simulink model "singleDPD"  (R2023a)
settings: Solver=FixedStepAuto  StartTime=0.0  StopTime=5*Tstep*ofdmSymLen*6  RelTol=1e-3
PreLoadFcn:
  | %{
  | % 100 MHz scenario
  | % scs = 30e3;
  | % fftLength = 4096;
  | % NSubcarriers = 3276;
  | % cpLength = 288;
  | % windowLength = 20;
  | 
  | % 5 MHz scenario
  | scs = 30e3;
  | fftLength = 256;
  | NSubcarriers = 132;
  | cpLength = 18;
  | windowLength = 6;
  | 
  | nGuardBandCarrier = fftLength - NSubcarriers;
  | ofdmSymLen = fftLength+cpLength;
  | overSamplingRate = 7;
  | filterLength = 6*70;
  | 
  | BW = scs*fftLength;                       %  Signal BW
  | Tstep = 1/BW;                   %  Simulation BW BB
  | RF = 3.7e9;                       %  RF center frequency
  | IF = 500e6;                          % IF frequency
  | dataRatePA = 1/BW;  % PA characterization sample time
  | N = nGuardBandCarrier/2;
  | HPF_cutoff = RF - 500e6;
  | 
  | bw = 5e6; %100e6;
  | [txWaveform, sampleRate] = helperPACharGenerateOFDM(bw);
  | 
  | dataFileName = sprintf("helperPACharSavedData%dMHz",bw/1e6);
  | load(dataFileName,"results")
  | paInput = results.InputWaveform;
  | paOutput = results.OutputWaveform;
  | modType = 'memPoly';
  | memLen = 5;
  | degLen = 5;
  | halfDataPts = round(length(paInput)/2);
  | origState = warning;
  | warning('off', 'MATLAB:rankDeficientMatrix')
  | paModelMemPoly = double(helperPACharMemPolyModel('coefficientFinder', ...
  |   paInput(1:halfDataPts),paOutput(1:halfDataPts),memLen,degLen,modType));
  | warning(origState);
  | 
  | gain = results.LinearGain;
  | scaleFactor = double(max(abs(paOutput))/max(abs(txWaveform))/gain);
  | %}
InitFcn:
  | % 100 MHz scenario
  |  scs = 30e3;
  |  fftLength = 4096;
  |  NSubcarriers = 3276;
  |  cpLength = 288;
  |  windowLength = 20;
  | 
  | % 5 MHz scenario
  | %scs = 30e3; % Subcarrier spacing
  | %fftLength = 256;
  | %NSubcarriers = 132;
  | %cpLength = 18; % cyclic prefix length
  | %windowLength = 6;
  | 
  | nGuardBandCarrier = fftLength - NSubcarriers;
  | ofdmSymLen = fftLength+cpLength;
  | overSamplingRate = 7;
  | filterLength = 6*70;
  | 
  | BW = scs*fftLength;                       %  Signal BW
  | Tstep = 1/BW;                   %  Simulation BW BB
  | RF = 1e9; %3.7e9;                       %  RF center frequency
  | IF = 500e6;                          % IF frequency
  | dataRatePA = 1/BW;  % PA characterization sample time
  | N = nGuardBandCarrier/2;
  | HPF_cutoff = RF - 500e6;
  | 
  | bw = 5e6; %100e6;
  | [txWaveform, sampleRate] = helperPACharGenerateOFDM(bw);
  | 
  | dataFileName = sprintf("helperPACharSavedData%dMHz",bw/1e6);
  | dataFileName = "helperPACharSavedData100MHz"
  | load(dataFileName,"results")
  | paInput = results.InputWaveform;
  | paOutput = results.OutputWaveform;
  | modType = 'memPoly';
  | memLen = 5;
  | degLen = 5;
  | halfDataPts = round(length(paInput)/2);
  | origState = warning;
  | warning('off', 'MATLAB:rankDeficientMatrix')
  | paModelMemPoly = double(helperPACharMemPolyModel('coefficientFinder', ...
  |   paInput(1:halfDataPts),paOutput(1:halfDataPts),memLen,degLen,modType));
  | warning(origState);
  | 
  | gain = results.LinearGain;
  | scaleFactor = double(max(abs(paOutput))/max(abs(txWaveform))/gain);
undefined symbols (not defined in the file or in its folder): hpaGain, S
libraries: simrfV2elements x20, simrfV2util1 x11, dspstat3 x8, simrfV2systems x3, simrfV2_lib x3, commofdm x2, simrfV2junction1 x2, commrfcorlib x2, simulink x2, commrandsrc3 x1, commdigbbndam3 x1, commutil2 x1
Description:
  | Power Amplifier Characterization with DPD for Reduced Signal Distortion
settings Model: SimulationMode=accelerator  Creator=The MathWorks, Inc.  LastModifiedBy=Hossein
settings SolverCC: ZeroCrossAlgorithm=Adaptive  AlgebraicLoopSolver=TrustRegion
settings DataIOCC: LimitDataPoints=on  SaveFormat=Array  SaveOutput=off  SignalLogging=off  DSMLogging=off  SaveTime=off  ReturnWorkspaceOutputs=off
settings OptimizationCC: BlockReduction=off  BooleanDataType=off  ReuseModelBlockBuffer=off  LifeSpan=inf
settings DebuggingCC: SaveWithParameterizedLinksMsg=none  UnderspecifiedInitializationDetection=Classic  MergeDetectMultiDrivingBlocksExec=none  SignalResolutionControl=TryResolveAllWithWarning  UnconnectedInputMsg=warning  UnconnectedOutputMsg=warning  UnconnectedLineMsg=warning  AllowSymbolicDim=off  SFUnexpectedBacktrackingDiag=warning  SFNoUnconditionalDefaultTransitionDiag=warning  SFExecutionAtInitializationDiag=none  ArithmeticOperatorsInVariantConditions=warning
settings HardwareCC: ProdBitPerPointer=32  ProdBitPerSizeT=32  ProdBitPerPtrDiffT=32  ProdLargestAtomicFloat=None  ProdIntDivRoundTo=Undefined  ProdEndianess=Unspecified  ProdWordSize=32  ProdHWDeviceType=32-bit Generic  TargetBitPerPointer=64  TargetBitPerSizeT=64  TargetBitPerPtrDiffT=64  TargetLongLongMode=on  TargetIntDivRoundTo=Zero  TargetEndianess=LittleEndian  TargetWordSize=64  TargetHWDeviceType=MATLAB Host  ProdEqTarget=off
settings ModelReferenceCC: EnableRefExpFcnMdlSchedulingChecks=on  PropagateSignalLabelsOutOfModel=off
settings SFSimCC: SimUseLocalCustomCode=off
settings RTWCC: RTWUseLocalCustomCode=off  BuildConfiguration=Faster Runs  DLArmComputeVersion=19.05
settings CodeAppCC: StateflowObjectComments=on
settings GRTTargetCC: TargetLangStandard=C89/C90 (ANSI)
settings ConfigComp: CovMetricSettings=dw  CovSaveCumulativeToWorkspaceVar=on  CovSaveSingleToWorkspaceVar=on  CovExternalEMLEnable=off
settings SimscapeCC: SimscapeNormalizeSystem=off

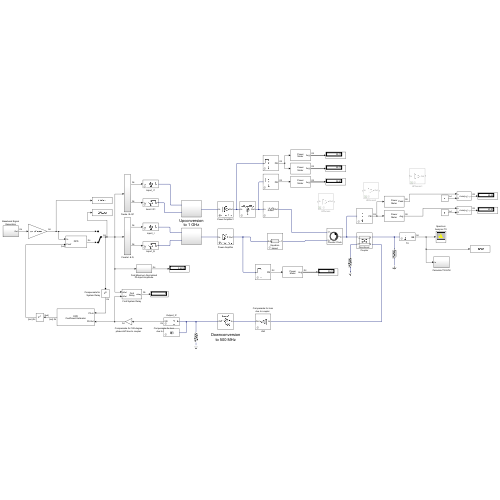
[thumbnail: Simulink's stored preview of the top-level diagram]
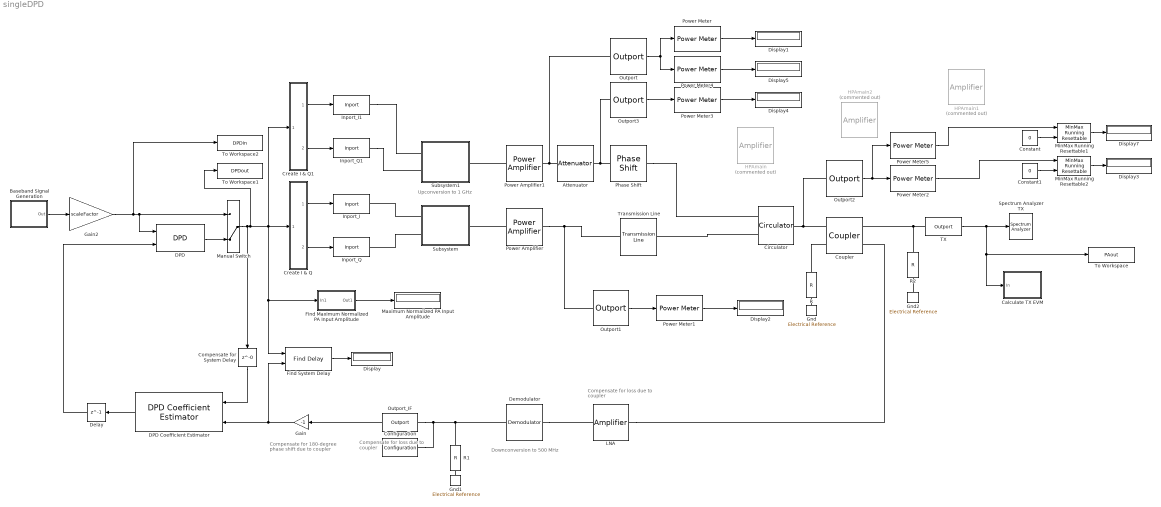
== system singleDPD ==
  note: Upconversion
      | to 1 GHz
  note: Compensate for loss
      | due to coupler
  note: Compensate for 180-degree
      | phase shift due to coupler
  note: Downconversion
      | to 500 MHz
  note: Compensate for loss
      | due to coupler
  Attenuator : simrfV2elements/Attenuator  classname=attenuator  Att=2.5  Zin=50  Zout=50  AddNoise=on  InternalGrounding=on
  Baseband Signal Generation : Subsystem
  Calculate TX EVM : Subsystem
  Circulator : simrfV2junction1/Circulator  classname=circulators  DataSource=Network-parameters  NumPorts=3  DeviceCirculator=Circulator counter clockwise  DeviceDivider=T power divider  DeviceCoupler=Directional coupler  Paramtype=S-parameters  Sparam=[0 0 1; 1 0 0; 0 1 0]  SparamFreq=1e9 Hz  SparamZ0=50  Phase12=0  Phase33=0  Alpha=0  NumberDividerOutports=2  Coupling=0  Directivity=inf  InsertionLoss=inf  ReturnLoss=inf  InternalGrounding=on  SparamRepresentation=Frequency domain  FitOpt=Share all poles  FitTol=-40  MaxPoles=48
  Compensate for System Delay : Delay  DelayLength=0
  Configuration : simrfV2util1/Configuration  AutoFreq=on  Tones="[3.2         3.7] GHz"  Harmonics="[5  5]"  NormalizeCarrierPower=on  SolverType=Auto  UseCCode=on  StepSize=Tstep/overSamplingRate s  AddNoise=on  defaultRNG=on  Seed=0  Temperature=290.0 K  SolverDelFlag=0  AbsTol=1e-6  RelTol=1e-3  MaxIter=10  ErrorEstimationType=2-norm over all variables  EnableInterpFilter=off  HiddenFIRfilterControllerParam=off  SmallSignalApprox=off  AllSimFreqs=on  SimFreqs=[] Hz  SimFreqsInternal=[]  SamplesPerFrame=1
  Constant : Constant  Value=0
  Constant1 : Constant  Value=0
  Coupler : simrfV2junction1/Coupler  classname=couplers  DataSource=Network-parameters  NumPorts=4  DeviceCirculator=Circulator clockwise  DeviceDivider=T power divider  DeviceCoupler=Directional coupler  Paramtype=S-parameters  Sparam=[0 0 1; 1 0 0; 0 1 0]  SparamFreq=1e9 Hz  SparamZ0=50  Phase12=0  Phase33=0  Alpha=0  NumberDividerOutports=2  Coupling=55  Directivity=inf  InsertionLoss=0.0001  ReturnLoss=inf  InternalGrounding=on  SparamRepresentation=Frequency domain  FitOpt=Share all poles  FitTol=-40  MaxPoles=48
  Create I & Q : Subsystem
  Create I & Q1 : Subsystem
  DPD : commrfcorlib/DPD  PolynomialType=Memory polynomial  CoefficientSource=Input port  Coefficients=complex([1 0 0 0 0; 0 0 0 0 0; 0 0 0 0 0])  SimulateUsing=Code generation
  DPD Coefficient Estimator : commrfcorlib/DPD Coefficient Estimator  DesiredAmplitudeGaindB=10*log10(gain)  PolynomialType=Memory polynomial  Degree=6  MemoryDepth=5  Algorithm=Recursive least squares  ForgettingFactorSource=Property  ForgettingFactor=0.999  InitialCoefficientEstimate=[]  SimulateUsing=Code generation
  Delay : Delay  DelayLength=1
  Demodulator : simrfV2systems/Demodulator  classname=rfdemod  Source_linear_gain=Available power gain  linear_gain=0 dB  Poly_Coeffs=[0 1]  LOFreq=RF-IF Hz  Zin=50  Zout=50  AddIRFilter=on  AddCSFilter=off  InternalGrounding=on  ForceNextInit=off  Source_Poly=Even and odd order  IPType=Input  IP2=inf dBm  IP3=inf dBm  P1dB=inf dBm  Psat=inf dBm  Gcomp=inf dBm  NF=1  Isolation=inf dB  AddPhaseNoise=off  PhaseNoiseOffset=[5e5 1e6 5e6]  PhaseNoiseLevel=[-108 -130 -140]  AutoImpulseLengthPN=on  ImpulseLengthPN=1e-10  ImpulseLength_unitPN=s  DesignMethodIR=Ideal  ResponseTypeIR=Highpass  ImplementationIR=LC Tee  ImplementationIdealIR=Constant per carrier  ImplementationRationalIR=Transfer function  UseFilterOrderIR=on  FilterOrderIR=3  PassFreq_lpIR=1  PassFreq_lp_unitIR=GHz  PassFreq_hpIR=HPF_cutoff  PassFreq_hp_unitIR=Hz  PassFreq_bpIR=[2 3]  PassFreq_bp_unitIR=GHz  PassFreq_bsIR=[1 4]  PassFreq_bs_unitIR=GHz  PassAttenIR=10*log10(2)  StopFreq_lpIR=2  StopFreq_lp_unitIR=GHz  StopFreq_hpIR=1  StopFreq_hp_unitIR=GHz  StopFreq_bpIR=[1.5 3.5]  StopFreq_bp_unitIR=GHz  StopFreq_bsIR=[2.1 2.9]  StopFreq_bs_unitIR=GHz  StopAttenIR=40  RsrcIR=50  RloadIR=50  AutoImpulseLengthIR=on  ImpulseLengthIR=1e-10  ImpulseLength_unitIR=s  DesignMethodCS=Ideal  ResponseTypeCS=Lowpass  ImplementationCS=LC Tee  ImplementationIdealCS=Constant per carrier  ImplementationRationalCS=Transfer function  UseFilterOrderCS=on  FilterOrderCS=3  PassFreq_lpCS=1  PassFreq_lp_unitCS=GHz  PassFreq_hpCS=2  PassFreq_hp_unitCS=GHz  PassFreq_bpCS=[2 3]  PassFreq_bp_unitCS=GHz  PassFreq_bsCS=[1 4]  PassFreq_bs_unitCS=GHz  PassAttenCS=10*log10(2)  StopFreq_lpCS=2  StopFreq_lp_unitCS=GHz  StopFreq_hpCS=1  StopFreq_hp_unitCS=GHz  StopFreq_bpCS=[1.5 3.5]  StopFreq_bp_unitCS=GHz  StopFreq_bsCS=[2.1 2.9]  StopFreq_bs_unitCS=GHz  StopAttenCS=40  RsrcCS=50  RloadCS=50  AutoImpulseLengthCS=on  ImpulseLengthCS=1e-10  ImpulseLength_unitCS=s
  Display{,1..5,7} (7 alike) : Display
  Find Maximum Normalized PA Input Amplitude : Subsystem
  Find System Delay : commutil2/Find Delay  corrLength=200  chgSigOP=off  stopUpdate=off  numConstDelay=3
  Gain : Gain  Gain=-1
  Gain2 : Gain  Gain=scaleFactor
  Gnd : simrfV2_lib/Elements/Electrical Reference
      settings: InternalSimscapePortConfiguration="{\"Bottom\":[],\"Left\":[{\"id\":\"V\",\"label\":\"\",\"type\":\"foundation.rf.circuitenvelope\"}],\"Right\":[],\"Top\":[]}"
  Gnd1 : simrfV2_lib/Elements/Electrical Reference
      settings: InternalSimscapePortConfiguration="{\"Bottom\":[],\"Left\":[{\"id\":\"V\",\"label\":\"\",\"type\":\"foundation.rf.circuitenvelope\"}],\"Right\":[],\"Top\":[]}"
  Gnd2 : simrfV2_lib/Elements/Electrical Reference
      settings: InternalSimscapePortConfiguration="{\"Bottom\":[],\"Left\":[{\"id\":\"V\",\"label\":\"\",\"type\":\"foundation.rf.circuitenvelope\"}],\"Right\":[],\"Top\":[]}"
  HPAmain : simrfV2elements/Amplifier  Commented=on  classname=amplifier  DataSource=Network-parameters  File=unitygain.s2p  isNetworkObj=off  Paramtype=S-parameters  Sparam=0  SparamFreq=CarrierFreq GHz  SparamZ0=50  isRationalObj=off  Residues=0  Poles=0  DF={0 0; 1 0}  Source_linear_gain=Available power gain  linear_gain=hpaGain - 3.5 dB  AmAmAmPmTable=[-25,5,-1;-10,20,-2;0,27,5;5,28,12]  Zin=50  Zout=50  Source_Poly=Odd order  Poly_Coeffs=[0 1]  IPType=Output  IP2=inf dBm  IP3=hpaIP3 dBm  P1dB=hpaP1dB dBm  Psat=inf dBm  Gcomp=inf dBm  InternalGrounding=on  SourceFreq=Extracted from data source  PlotFreq=1 Hz  PlotType=X-Y plane  YParam1=S(2,1)  YFormat1=Magnitude (dB)  YParam2=None  YFormat2=Magnitude (dB)  YOption=Linear  XOption=Linear  SparamRepresentation=Frequency domain  FitTol=-40  FitOpt=Fit individually  MaxPoles=48  AutoImpulseLength=off  ImpulseLength=0 s  MagModeling=off  AddNoise=on  NoiseType=Noise figure  NoiseDist=White  NF=hpaNF  MinNF=0  Gopt=0  RN=0  CarrierFreq=0 Hz  NoiseAutoImpulseLength=on  NoiseImpulseLength=1e-10 s  ConstS21NL=on  OpFreq=0 Hz  SetOpFreqAsMaxS21=on
  HPAmain1 : simrfV2elements/Amplifier  Commented=on  classname=amplifier  DataSource=Network-parameters  File=unitygain.s2p  isNetworkObj=off  Paramtype=S-parameters  Sparam=0  SparamFreq=CarrierFreq GHz  SparamZ0=50  isRationalObj=off  Residues=0  Poles=0  DF={0 0; 1 0}  Source_linear_gain=Available power gain  linear_gain=10 dB  AmAmAmPmTable=[-25,5,-1;-10,20,-2;0,27,5;5,28,12]  Zin=50  Zout=50  Source_Poly=Odd order  Poly_Coeffs=[0 1]  IPType=Output  IP2=inf dBm  IP3=48 dBm  P1dB=40 dBm  Psat=45 dBm  Gcomp=inf dBm  InternalGrounding=on  SourceFreq=Extracted from data source  PlotFreq=1 Hz  PlotType=X-Y plane  YParam1=S(2,1)  YFormat1=Magnitude (dB)  YParam2=None  YFormat2=Magnitude (dB)  YOption=Linear  XOption=Linear  SparamRepresentation=Frequency domain  FitTol=-40  FitOpt=Fit individually  MaxPoles=48  AutoImpulseLength=off  ImpulseLength=0 s  MagModeling=off  AddNoise=on  NoiseType=Noise figure  NoiseDist=White  NF=0  MinNF=0  Gopt=0  RN=0  CarrierFreq=0 Hz  NoiseAutoImpulseLength=on  NoiseImpulseLength=1e-10 s  ConstS21NL=on  OpFreq=0 Hz  SetOpFreqAsMaxS21=on
  HPAmain2 : simrfV2elements/Amplifier  Commented=on  classname=amplifier  DataSource=Network-parameters  File=unitygain.s2p  isNetworkObj=off  Paramtype=S-parameters  Sparam=0  SparamFreq=CarrierFreq GHz  SparamZ0=50  isRationalObj=off  Residues=0  Poles=0  DF={0 0; 1 0}  Source_linear_gain=Available power gain  linear_gain=10 dB  AmAmAmPmTable=[-25,5,-1;-10,20,-2;0,27,5;5,28,12]  Zin=50  Zout=50  Source_Poly=Odd order  Poly_Coeffs=[0 1]  IPType=Output  IP2=inf dBm  IP3=48 - 3.5 dBm  P1dB=40 - 3.5 dBm  Psat=45 - 3.5 dBm  Gcomp=inf dBm  InternalGrounding=on  SourceFreq=Extracted from data source  PlotFreq=1 Hz  PlotType=X-Y plane  YParam1=S(2,1)  YFormat1=Magnitude (dB)  YParam2=None  YFormat2=Magnitude (dB)  YOption=Linear  XOption=Linear  SparamRepresentation=Frequency domain  FitTol=-40  FitOpt=Fit individually  MaxPoles=48  AutoImpulseLength=off  ImpulseLength=0 s  MagModeling=off  AddNoise=on  NoiseType=Noise figure  NoiseDist=White  NF=0  MinNF=0  Gopt=0  RN=0  CarrierFreq=0 Hz  NoiseAutoImpulseLength=on  NoiseImpulseLength=1e-10 s  ConstS21NL=on  OpFreq=0 Hz  SetOpFreqAsMaxS21=on
  Inport_I : simrfV2util1/Inport  SimulinkInputSignalType=Ideal voltage  CarrierFreq=0 Hz  ZS=0  UseSqWave=off  NumCoeff=10  Bias=0  DutyCyc=50  InternalGrounding=on
  Inport_I1 : simrfV2util1/Inport  SimulinkInputSignalType=Ideal voltage  CarrierFreq=0 Hz  ZS=0  UseSqWave=off  NumCoeff=10  Bias=0  DutyCyc=50  InternalGrounding=on
  Inport_Q : simrfV2util1/Inport  SimulinkInputSignalType=Ideal voltage  CarrierFreq=0 Hz  ZS=0  UseSqWave=off  NumCoeff=10  Bias=0  DutyCyc=50  InternalGrounding=on
  Inport_Q1 : simrfV2util1/Inport  SimulinkInputSignalType=Ideal voltage  CarrierFreq=0 Hz  ZS=0  UseSqWave=off  NumCoeff=10  Bias=0  DutyCyc=50  InternalGrounding=on
  LNA : simrfV2elements/Amplifier  classname=amplifier  DataSource=Data file  File=unitygain.s2p  isNetworkObj=off  Paramtype=S-parameters  Sparam=[0 0;1 0]  SparamFreq=1e9 Hz  SparamZ0=50  isRationalObj=off  Residues=0  Poles=0  DF={0 0; 1 0}  Source_linear_gain=Available power gain  linear_gain=55 dB  AmAmAmPmTable=[-25,5,-1;-10,20,-2;0,27,5;5,28,12]  Zin=50  Zout=50  Source_Poly=Odd order  Poly_Coeffs=[0 1]  IPType=Output  IP2=19.5 dBm  IP3=inf dBm  P1dB=inf dBm  Psat=inf dBm  Gcomp=inf dBm  InternalGrounding=on  SourceFreq=Extracted from data source  PlotFreq=0 Hz  PlotType=X-Y plane  YParam1=S(1,1)  YFormat1=Magnitude (dB)  YParam2=None  YFormat2=Magnitude (dB)  YOption=Linear  XOption=Linear  SparamRepresentation=Time domain (rationalfit)  FitTol=-40  FitOpt=Share all poles  MaxPoles=48  AutoImpulseLength=off  ImpulseLength=0 s  MagModeling=off  AddNoise=on  NoiseType=Noise figure  NoiseDist=White  NF=0.1  MinNF=0  Gopt=0  RN=0  CarrierFreq=0 Hz  NoiseAutoImpulseLength=on  NoiseImpulseLength=1e-10 s  ConstS21NL=on  OpFreq=0 Hz  SetOpFreqAsMaxS21=on
  Manual Switch : ManualSwitch  CurrentSetting=0
  Maximum Normalized PA Input Amplitude : Display
  MinMax Running Resettable1 : simulink/Math Operations/MinMax Running Resettable  Function=max  vinit=0.0
  MinMax Running Resettable2 : simulink/Math Operations/MinMax Running Resettable  Function=max  vinit=0.0
  Outport{,1..3} (4 alike) : simrfV2util1/Outport  SensorType=Ideal voltage  OutputFormat=Real Passband  CarrierFreq=RF Hz  ZL=Inf  InternalGrounding=on  StepSize=1e-6 s  AutoStep=on  HalfPolyphaseLength=12
  Outport_IF : simrfV2util1/Outport  SensorType=Ideal voltage  OutputFormat=Complex Baseband  CarrierFreq=IF Hz  ZL=Inf  InternalGrounding=on  StepSize=-1 s  AutoStep=off  HalfPolyphaseLength=0
  Phase Shift : simrfV2elements/Phase Shift  PhaseShift=90 deg  InternalGrounding=on
  Power Amplifier : simrfV2elements/Power Amplifier  classname=poweramp  ModelType=Memory polynomial  CoeffMatrix=paModelMemPoly  UnitDelay=dataRatePA/overSamplingRate  Rin=50  Rout=50  InternalGrounding=on
  Power Amplifier1 : simrfV2elements/Power Amplifier  classname=poweramp  ModelType=Memory polynomial  CoeffMatrix=paModelMemPoly  UnitDelay=dataRatePA/overSamplingRate  Rin=50  Rout=50  InternalGrounding=on
  Power Meter{,1,3..4} (4 alike) : dspstat3/Power Meter  Measurement=Average power  ReferenceLoad=50  OutputPowerUnits=dBm  WindowLength=2048  OverlapLength=2047  AllowArbitraryInputLength=on  ComputeCCDF=off  PowerRange=50  PowerResolution=0.1  CCDFOutput=Relative power (dB above average power)  ProbabilityVector=[ 10; 1; 0.1; 0.01; 0.001; 0.0001 ]  RelativePowerVector=[ 0; 3; 6; 9; 12 ]  ResetPort=off  SimulateUsing=Code generation
      settings: LibrarySourceBlock=commutil2/Power Meter
  Power Meter2 : dspstat3/Power Meter  Measurement=Average power  ReferenceLoad=50  OutputPowerUnits=dBm  WindowLength=2048*2  OverlapLength=2047*2+1  AllowArbitraryInputLength=off  ComputeCCDF=off  PowerRange=50  PowerResolution=0.1  CCDFOutput=Relative power (dB above average power)  ProbabilityVector=[ 10; 1; 0.1; 0.01; 0.001; 0.0001 ]  RelativePowerVector=[ 0; 3; 6; 9; 12 ]  ResetPort=off  SimulateUsing=Code generation
      settings: LibrarySourceBlock=commutil2/Power Meter
  Power Meter5 : dspstat3/Power Meter  Measurement=Peak power  ReferenceLoad=50  OutputPowerUnits=dBm  WindowLength=2048*2  OverlapLength=2047*2+1  AllowArbitraryInputLength=off  ComputeCCDF=off  PowerRange=50  PowerResolution=0.1  CCDFOutput=Relative power (dB above average power)  ProbabilityVector=[ 10; 1; 0.1; 0.01; 0.001; 0.0001 ]  RelativePowerVector=[ 0; 3; 6; 9; 12 ]  ResetPort=off  SimulateUsing=Code generation
      settings: LibrarySourceBlock=commutil2/Power Meter
  R : simrfV2elements/R  classname=resistor  Resistance=50 Ohm  AddNoise=on
  R1 : simrfV2elements/R  classname=resistor  Resistance=50 Ohm  AddNoise=on
  R2 : simrfV2elements/R  classname=resistor  Resistance=50 Ohm  AddNoise=on
  Spectrum Analyzer TX : SpectrumAnalyzer  WindowPosition=[962.000000,50.000000,958.000000,1000.000000,]  Visible=on  ScopeFrameLocation=window  SampleRate=860160000  AxesScaling=Manual  Span=1843200000  StartFrequency=-921600000  StopFrequency=921600000  FrequencyResolutionMethod=Window length  WindowLength=8192  AveragingMethod=Running  SpectralAverages=4  ReferenceLoad=50  YLimits=[-76.29372752,28.83162013]  ExpandToolstrip=on  DefaultConfigurationName=spbscopes.SpectrumAnalyzerBlockCfg  IsFrequencyInputMode=0  FrequencyVectorPort=0  FrequencyVectorFromPort=0  FrequencyInputRBWPort=0  FrequencyInputRBWFromPort=0
  Subsystem : Subsystem
  Subsystem1 : Subsystem
  TX : simrfV2util1/Outport  SensorType=Ideal voltage  OutputFormat=Complex Baseband  CarrierFreq=RF Hz  ZL=Inf  InternalGrounding=on  StepSize=-1 s  AutoStep=off  HalfPolyphaseLength=0
  To Workspace : ToWorkspace  VariableName=PAout  SampleTime=-1
      settings: Save2DSignal=2-D array (concatenate along first dimension)
  To Workspace1 : ToWorkspace  VariableName=DPDout  SampleTime=-1
      settings: Save2DSignal=2-D array (concatenate along first dimension)
  To Workspace2 : ToWorkspace  VariableName=DPDin  SampleTime=-1
      settings: Save2DSignal=2-D array (concatenate along first dimension)
  Transmission Line : simrfV2elements/Transmission Line  classname=xline  Model_type=Equation-based  ConductorBacked=off  StructureMicrostrip=Standard  Parameterization=By characteristic impedance and capacitance  TransDelay=4.7e-9 s  CharImped=25 Ohm  Resistance=0.3 Ohm/m  Inductance=235e-9 H/m  Capacitance=94e-12 F/m  Conductance=5e-6 S/m  LineLength=(3e8/1e9)/4 m  NumSegments=10  InternalGrounding=on  OuterRadius=2.57 mm  InnerRadius=0.725 mm  MuR=1  EpsilonR=2.2  LossTangent=0  SigmaCond=inf S/m  StubMode=Not a stub  Termination=Open  ConductorWidth=0.6 mm  SlotWidth=0.2 mm  Height=0.635 mm  Height_inv=0.635 mm  Height_spd=0.3175 mm  Height_emb=1.37 mm  StripHeight=0.635 mm  Thickness=5 um  SWidth=0.6 mm  Radius=0.67 mm  Separation=1.62 mm  PWidth=5 mm  PSeparation=1 mm  PV=3e8  Loss=0  SourceFreq=User-specified  PlotFreq=[0.9e9:0.5e6:1.1e9] Hz  PlotType=X-Y plane  YParam1=S(2,1)  YFormat1=Angle (degrees)  YParam2=none  YFormat2=Magnitude (dB)  YOption=Linear  XOption=Linear  FitOpt=Share all poles  FitTol=-40  MaxPoles=48  SparamRepresentation=Frequency domain  Freq=1 Ghz  Interp_type=Linear  AutoImpulseLength=off  ImpulseLength=0 s  MagModeling=off
  wires:
  DPD/1 -> Manual Switch/2
  DPD Coefficient Estimator/1 -> Delay/1
  Delay/1 -> DPD/2
  Find System Delay/1 -> Display/1
  Compensate for System Delay/1 -> DPD Coefficient Estimator/1
  Create I & Q/1(Out1) -> Inport_I/1
  Create I & Q/2(Out2) -> Inport_Q/1
  Gain/1 -> Find System Delay/2, DPD Coefficient Estimator/2
  Outport_IF/1 -> Gain/1
  Baseband Signal Generation/1(Out) -> Gain2/1
  TX/1 -> Calculate TX EVM/1(In), To Workspace/1, Spectrum Analyzer TX/1
  Manual Switch/1 -> Compensate for System Delay/1, To Workspace1/1, Create I & Q1/1(In1), Find System Delay/1, Find Maximum Normalized PA Input Amplitude/1(In1), Create I & Q/1(In1)
  Find Maximum Normalized PA Input Amplitude/1(Out1) -> Maximum Normalized PA Input Amplitude/1
  Gain2/1 -> To Workspace2/1, DPD/1, Manual Switch/1
  Create I & Q1/2(Out2) -> Inport_Q1/1
  Create I & Q1/1(Out1) -> Inport_I1/1
  Power Meter/1 -> Display1/1
  Power Meter1/1 -> Display2/1
  Outport1/1 -> Power Meter1/1
  Outport2/1 -> Power Meter5/1, Power Meter2/1
  Power Meter3/1 -> Display4/1
  Outport3/1 -> Power Meter3/1
  Power Meter4/1 -> Display5/1
  Outport/1 -> Power Meter4/1, Power Meter/1
  MinMax Running Resettable1/1 -> Display7/1
  Constant/1 -> MinMax Running Resettable1/2
  Power Meter5/1 -> MinMax Running Resettable1/1
  Constant1/1 -> MinMax Running Resettable2/2
  MinMax Running Resettable2/1 -> Display3/1
  Power Meter2/1 -> MinMax Running Resettable2/1
  connections:
  TX/LConn1 -- Coupler/RConn1 -- R2/LConn1
  LNA/LConn1 -- Coupler/RConn2
  R/LConn1 -- Coupler/LConn2
  Demodulator/LConn1 -- LNA/RConn1
  Gnd/LConn1 -- R/RConn1
  Outport_IF/LConn1 -- R1/LConn1 -- Demodulator/RConn1 -- Configuration/LConn1
  Gnd1/LConn1 -- R1/RConn1
  Subsystem/LConn1 -- Inport_I/RConn1
  Power Amplifier/LConn1 -- Subsystem/RConn1
  Subsystem/LConn2 -- Inport_Q/RConn1
  Circulator/LConn2 -- Transmission Line/LConn1
  Circulator/RConn1 -- Outport2/LConn1 -- Coupler/LConn1
  Power Amplifier1/LConn1 -- Subsystem1/RConn1
  Inport_I1/RConn1 -- Subsystem1/LConn1
  Inport_Q1/RConn1 -- Subsystem1/LConn2
  Power Amplifier1/RConn1 -- Outport/LConn1 -- Attenuator/LConn1
  Attenuator/RConn1 -- Outport3/LConn1 -- Phase Shift/LConn1
  Power Amplifier/RConn1 -- Outport1/LConn1 -- Transmission Line/RConn1
  Gnd2/LConn1 -- R2/RConn1
  Phase Shift/RConn1 -- Circulator/LConn1

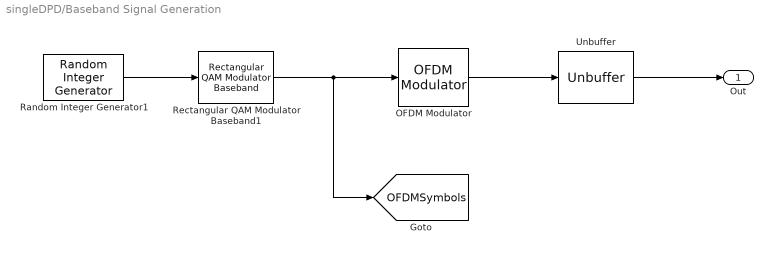
== system singleDPD/Baseband Signal Generation ==
  OFDM Modulator : commofdm/OFDM Modulator  FFTLength=fftLength  NumGuardBandCarriers=[N+1; N]  InsertDCNull=off  PilotInputPort=off  PilotCarrierIndices=[12; 26; 40; 54]  CyclicPrefixLength=cpLength  Windowing=on  WindowLength=windowLength  OversamplingFactor=overSamplingRate  NumSymbols=1  NumTransmitAntennas=1  SimulateUsing=Code generation
  Random Integer Generator1 : commrandsrc3/Random Integer Generator  SetSize=64  SeedSource=Parameter  Seed=242  SampleTime=Tstep*(ofdmSymLen/(fftLength-2*N-1))  SamplesPerFrame=fftLength-2*N-1  OutputDataType=double  SimulateUsing=Code generation
  Rectangular QAM Modulator Baseband1 : commdigbbndam3/Rectangular QAM Modulator Baseband  M=64  InType=Integer  Enc=Gray  Mapping=[0:15]  PowType=Min. distance between symbols  MinDist=2  AvgPow=1  PeakPow=1  Ph=0  outDtype=double  outWordLen=16  outUDDataType=sfix(16)  outFracLenMode=Best precision  outFracLen=15  outDataTypeStr=double  outLastDataTypeStr=double
  Unbuffer : Unbuffer
  Out : Outport  VectorParamsAs1DForOutWhenUnconnected=off
  tag scope: OFDMSymbols=global
  wires:
  Random Integer Generator1/1 -> Rectangular QAM Modulator Baseband1/1
  Unbuffer/1 -> Out/1
  Rectangular QAM Modulator Baseband1/1 -> [OFDMSymbols], OFDM Modulator/1
  OFDM Modulator/1 -> Unbuffer/1

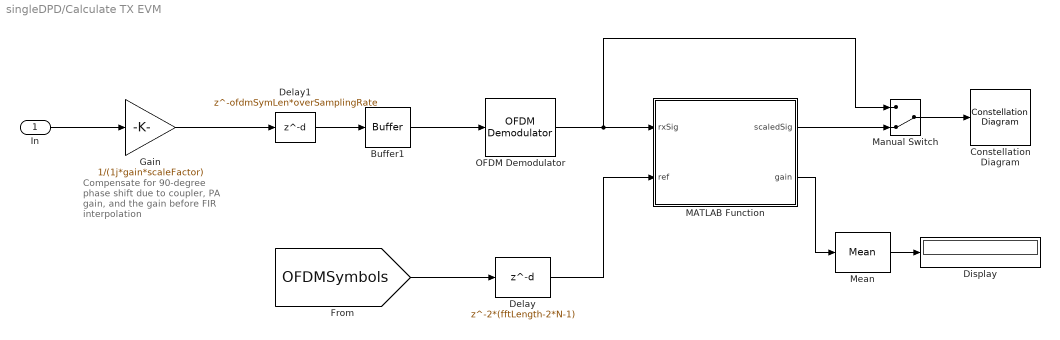
== system singleDPD/Calculate TX EVM ==
  note: Compensate for 90-degree
      | phase shift due to coupler,
      | PA gain, and the gain before
      | FIR interpolation
  In : Inport
  Buffer1 : Buffer  N=ofdmSymLen*overSamplingRate  OutputFrames=off
  Constellation Diagram : ConstellationDiagram  WindowPosition=[962.000000,50.000000,958.000000,1000.000000,]  ScopeFrameLocation=window  ReferenceConstellation="{[-7+7i  -7+5i  -7+3i  -7+1i  -7-1i  -7-3i  -7-5i  -7-7i  -5+7i  -5+5i  -5+3i  -5+1i  -5-1i  -5-3i  -5-5i  -5-7i  -3+7i  -3+5i  -3+3i  -3+1i  -3-1i  -3-3i  -3-5i  -3-7i  -1+7i  -1+5i  -1+3i  -1+1i  -1-1i  -1-3i  -1-5i  -1-7i   1+7i   1+5i   1+3i   1+1i   1-1i   1-3i   1-5i   1-7i   3+7i   3+5i   3+3i   3+1i   3-1i   3-3i   3-5i   3-7i   5+7i   5+5i   5+3i   5+1i   5-1i   5-3i   5-5i   5-7i   7+7i   7+5i   7+3i   7+1i   7-1i   7-3i   7-5i   7-7i]}"  XLimits=[-9.7559 9.963]  YLimits=[-9.7559 9.963]  EnableMeasurements=on  DefaultConfigurationName=comm.scopes.ConstellationDiagramBlockCfg
  Delay : Delay  DelayLength=2*(fftLength-2*N-1)  InputProcessing=Columns as channels (frame based)
  Delay1 : Delay  DelayLength=ofdmSymLen*overSamplingRate  InputProcessing=Columns as channels (frame based)
  Display : Display
  Gain : Gain  Gain=1/(1j*gain*scaleFactor)
  MATLAB Function : MATLAB Function  TreatAsAtomicUnit=on
  Manual Switch : ManualSwitch  CurrentSetting=0
  Mean : dspstat3/Mean  run=off  InputProcessing=Columns as channels (frame based)  reset_popup=None  directionMode=Each column  dimension=1  roiEnable=off  roiType=Rectangles  roiPortion=Entire ROI  roiOutput=Individual statistics for each ROI  roiFlag=off  roundingMode=Floor  overflowMode=off  outputDataTypeStr=Inherit: Same as accumulator  outputMin=[]  outputMax=[]  outputLastDataTypeStr=Inherit: Same as accumulator
  OFDM Demodulator : commofdm/OFDM Demodulator  FFTLength=fftLength  NumGuardBandCarriers=[N+1; N]  RemoveDCCarrier=off  PilotOutputPort=off  PilotCarrierIndices=[12; 26; 40; 54]  CyclicPrefixLength=cpLength  OversamplingFactor=overSamplingRate  NumSymbols=1  NumReceiveAntennas=1  SimulateUsing=Code generation
  wires:
  Buffer1/1 -> OFDM Demodulator/1
  In/1 -> Gain/1
  MATLAB Function/2(gain) -> Mean/1
  MATLAB Function/1(scaledSig) -> Manual Switch/2
  Manual Switch/1 -> Constellation Diagram/1
  OFDM Demodulator/1 -> MATLAB Function/1(rxSig), Manual Switch/1
  [OFDMSymbols] -> Delay/1
  Delay/1 -> MATLAB Function/2(ref)
  Mean/1 -> Display/1
  Gain/1 -> Delay1/1
  Delay1/1 -> Buffer1/1

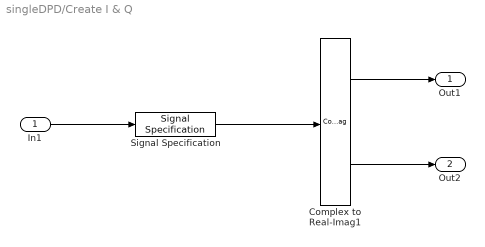
== system singleDPD/Create I & Q ==
  In1 : Inport
  Complex to Real-Imag1 : ComplexToRealImag
  Signal Specification : SignalSpecification  Dimensions=1
  Out1 : Outport  VectorParamsAs1DForOutWhenUnconnected=off
  Out2 : Outport  Port=2  VectorParamsAs1DForOutWhenUnconnected=off
  wires:
  Complex to Real-Imag1/1 -> Out1/1
  Complex to Real-Imag1/2 -> Out2/1
  In1/1 -> Signal Specification/1
  Signal Specification/1 -> Complex to Real-Imag1/1

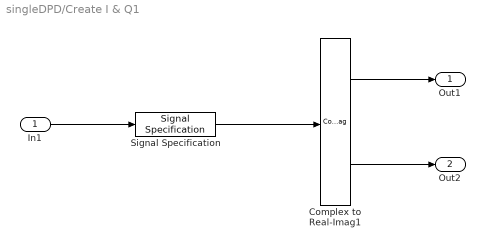
== system singleDPD/Create I & Q1 ==
  In1 : Inport
  Complex to Real-Imag1 : ComplexToRealImag
  Signal Specification : SignalSpecification  Dimensions=1
  Out1 : Outport  VectorParamsAs1DForOutWhenUnconnected=off
  Out2 : Outport  Port=2  VectorParamsAs1DForOutWhenUnconnected=off
  wires:
  Complex to Real-Imag1/1 -> Out1/1
  Complex to Real-Imag1/2 -> Out2/1
  In1/1 -> Signal Specification/1
  Signal Specification/1 -> Complex to Real-Imag1/1

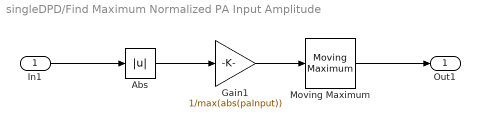
== system singleDPD/Find Maximum Normalized PA Input Amplitude ==
  In1 : Inport
  Abs : Abs  SaturateOnIntegerOverflow=off
  Gain1 : Gain  Gain=1/max(abs(paInput))
  Moving Maximum : dspstat3/Moving Maximum  SpecifyWindowLength=off  WindowLength=4  SimulateUsing=Code generation
  Out1 : Outport
  wires:
  Abs/1 -> Gain1/1
  Gain1/1 -> Moving Maximum/1
  Moving Maximum/1 -> Out1/1
  In1/1 -> Abs/1

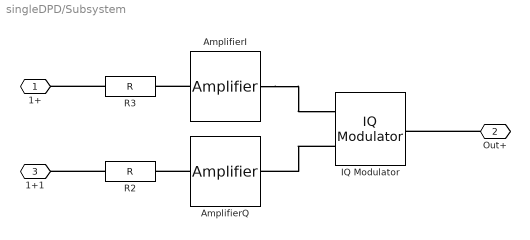
== system singleDPD/Subsystem ==
  AmplifierI : simrfV2elements/Amplifier  classname=amplifier  DataSource=Data file  File=unitygain.s2p  isNetworkObj=off  Paramtype=S-parameters  Sparam=[0 0;1 0]  SparamFreq=1e9 Hz  SparamZ0=50  isRationalObj=off  Residues=0  Poles=0  DF={0 0; 1 0}  Source_linear_gain=Available power gain  linear_gain=10*log10(4) dB  AmAmAmPmTable=[-25,5,-1;-10,20,-2;0,27,5;5,28,12]  Zin=50  Zout=50  Source_Poly=Even and odd order  Poly_Coeffs=[0 1]  IPType=Input  IP2=inf dBm  IP3=inf dBm  P1dB=inf dBm  Psat=inf dBm  Gcomp=inf dBm  InternalGrounding=on  SourceFreq=Extracted from data source  PlotFreq=[1e9:1e6:3e9] Hz  PlotType=X-Y plane  YParam1=S(1,1)  YFormat1=Magnitude (dB)  YParam2=None  YFormat2=Magnitude (dB)  YOption=Linear  XOption=Linear  SparamRepresentation=Time domain (rationalfit)  FitTol=-40  FitOpt=Fit individually  MaxPoles=48  AutoImpulseLength=on  ImpulseLength=1e-10 s  MagModeling=off  AddNoise=on  NoiseType=Noise figure  NoiseDist=White  NF=0.2  MinNF=0  Gopt=0  RN=0  CarrierFreq=0 Hz  NoiseAutoImpulseLength=on  NoiseImpulseLength=1e-10 s  ConstS21NL=on  OpFreq=0 Hz  SetOpFreqAsMaxS21=on
  AmplifierQ : simrfV2elements/Amplifier  classname=amplifier  DataSource=Data file  File=unitygain.s2p  isNetworkObj=off  Paramtype=S-parameters  Sparam=[0 0;1 0]  SparamFreq=1e9 Hz  SparamZ0=50  isRationalObj=off  Residues=0  Poles=0  DF={0 0; 1 0}  Source_linear_gain=Available power gain  linear_gain=10*log10(4) dB  AmAmAmPmTable=[-25,5,-1;-10,20,-2;0,27,5;5,28,12]  Zin=50  Zout=50  Source_Poly=Even and odd order  Poly_Coeffs=[0 1]  IPType=Input  IP2=inf dBm  IP3=inf dBm  P1dB=inf dBm  Psat=inf dBm  Gcomp=inf dBm  InternalGrounding=on  SourceFreq=Extracted from data source  PlotFreq=[1e9:1e6:3e9] Hz  PlotType=X-Y plane  YParam1=S(1,1)  YFormat1=Magnitude (dB)  YParam2=None  YFormat2=Magnitude (dB)  YOption=Linear  XOption=Linear  SparamRepresentation=Time domain (rationalfit)  FitTol=-40  FitOpt=Fit individually  MaxPoles=48  AutoImpulseLength=on  ImpulseLength=1e-10 s  MagModeling=off  AddNoise=on  NoiseType=Noise figure  NoiseDist=White  NF=0.2  MinNF=0  Gopt=0  RN=0  CarrierFreq=0 Hz  NoiseAutoImpulseLength=on  NoiseImpulseLength=1e-10 s  ConstS21NL=on  OpFreq=0 Hz  SetOpFreqAsMaxS21=on
  IQ Modulator : simrfV2systems/IQ Modulator  classname=iqmod  Source_linear_gain=Available power gain  linear_gain=10*log10(2) dB  Poly_Coeffs=[0 1]  LOFreq=RF Hz  Zin=50  Zout=50  AddIRFilters=off  AddCSFilter=on  InternalGrounding=on  ForceNextInit=off  NFloor=-inf  GainMismatch=0 dB  PhaseMismatch=0 deg  Isolation=inf dB  AddPhaseNoise=off  PhaseNoiseOffset=1e6  PhaseNoiseLevel=-140  AutoImpulseLengthPN=on  ImpulseLengthPN=1e-10  ImpulseLength_unitPN=s  Source_Poly=Even and odd order  IPType=Input  IP2=inf dBm  IP3=inf dBm  P1dB=inf dBm  Psat=inf dBm  Gcomp=inf dBm  DesignMethodIR=Ideal  ResponseTypeIR=Lowpass  ImplementationIR=LC Tee  ImplementationIdealIR=Constant per carrier  ImplementationRationalIR=Transfer function  UseFilterOrderIR=on  FilterOrderIR=3  PassFreq_lpIR=1  PassFreq_lp_unitIR=GHz  PassFreq_hpIR=2  PassFreq_hp_unitIR=GHz  PassFreq_bpIR=[2 3]  PassFreq_bp_unitIR=GHz  PassFreq_bsIR=[1 4]  PassFreq_bs_unitIR=GHz  PassAttenIR=10*log10(2)  StopFreq_lpIR=2  StopFreq_lp_unitIR=GHz  StopFreq_hpIR=1  StopFreq_hp_unitIR=GHz  StopFreq_bpIR=[1.5 3.5]  StopFreq_bp_unitIR=GHz  StopFreq_bsIR=[2.1 2.9]  StopFreq_bs_unitIR=GHz  StopAttenIR=40  RsrcIR=50  RloadIR=50  AutoImpulseLengthIR=on  ImpulseLengthIR=1e-10  ImpulseLength_unitIR=s  DesignMethodCS=Ideal  ResponseTypeCS=Highpass  ImplementationCS=LC Tee  ImplementationIdealCS=Constant per carrier  ImplementationRationalCS=Transfer function  UseFilterOrderCS=on  FilterOrderCS=3  PassFreq_lpCS=1  PassFreq_lp_unitCS=GHz  PassFreq_hpCS=HPF_cutoff  PassFreq_hp_unitCS=Hz  PassFreq_bpCS=[2 3]  PassFreq_bp_unitCS=GHz  PassFreq_bsCS=[1 4]  PassFreq_bs_unitCS=GHz  PassAttenCS=10*log10(2)  StopFreq_lpCS=2  StopFreq_lp_unitCS=GHz  StopFreq_hpCS=1  StopFreq_hp_unitCS=GHz  StopFreq_bpCS=[1.5 3.5]  StopFreq_bp_unitCS=GHz  StopFreq_bsCS=[2.1 2.9]  StopFreq_bs_unitCS=GHz  StopAttenCS=40  RsrcCS=50  RloadCS=50  AutoImpulseLengthCS=on  ImpulseLengthCS=1e-10  ImpulseLength_unitCS=s
  R2 : simrfV2elements/R  classname=resistor  Resistance=50 Ohm  AddNoise=on
  R3 : simrfV2elements/R  classname=resistor  Resistance=50 Ohm  AddNoise=on
  1+ : PMIOPort  Side=Left
  Out+ : PMIOPort  Port=2  Side=Right
  1+1 : PMIOPort  Port=3  Side=Left
  connections:
  Out+/RConn1 -- IQ Modulator/RConn1
  IQ Modulator/LConn2 -- AmplifierQ/RConn1
  AmplifierI/LConn1 -- R3/RConn1
  AmplifierI/RConn1 -- IQ Modulator/LConn1
  R3/LConn1 -- 1+/RConn1
  AmplifierQ/LConn1 -- R2/RConn1
  R2/LConn1 -- 1+1/RConn1

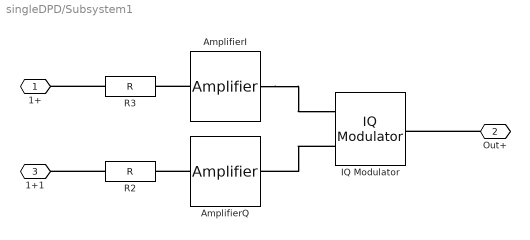
== system singleDPD/Subsystem1 ==
  AmplifierI : simrfV2elements/Amplifier  classname=amplifier  DataSource=Data file  File=unitygain.s2p  isNetworkObj=off  Paramtype=S-parameters  Sparam=[0 0;1 0]  SparamFreq=1e9 Hz  SparamZ0=50  isRationalObj=off  Residues=0  Poles=0  DF={0 0; 1 0}  Source_linear_gain=Available power gain  linear_gain=10*log10(4) dB  AmAmAmPmTable=[-25,5,-1;-10,20,-2;0,27,5;5,28,12]  Zin=50  Zout=50  Source_Poly=Even and odd order  Poly_Coeffs=[0 1]  IPType=Input  IP2=inf dBm  IP3=inf dBm  P1dB=inf dBm  Psat=inf dBm  Gcomp=inf dBm  InternalGrounding=on  SourceFreq=Extracted from data source  PlotFreq=[1e9:1e6:3e9] Hz  PlotType=X-Y plane  YParam1=S(1,1)  YFormat1=Magnitude (dB)  YParam2=None  YFormat2=Magnitude (dB)  YOption=Linear  XOption=Linear  SparamRepresentation=Time domain (rationalfit)  FitTol=-40  FitOpt=Fit individually  MaxPoles=48  AutoImpulseLength=on  ImpulseLength=1e-10 s  MagModeling=off  AddNoise=on  NoiseType=Noise figure  NoiseDist=White  NF=0.2  MinNF=0  Gopt=0  RN=0  CarrierFreq=0 Hz  NoiseAutoImpulseLength=on  NoiseImpulseLength=1e-10 s  ConstS21NL=on  OpFreq=0 Hz  SetOpFreqAsMaxS21=on
  AmplifierQ : simrfV2elements/Amplifier  classname=amplifier  DataSource=Data file  File=unitygain.s2p  isNetworkObj=off  Paramtype=S-parameters  Sparam=[0 0;1 0]  SparamFreq=1e9 Hz  SparamZ0=50  isRationalObj=off  Residues=0  Poles=0  DF={0 0; 1 0}  Source_linear_gain=Available power gain  linear_gain=10*log10(4) dB  AmAmAmPmTable=[-25,5,-1;-10,20,-2;0,27,5;5,28,12]  Zin=50  Zout=50  Source_Poly=Even and odd order  Poly_Coeffs=[0 1]  IPType=Input  IP2=inf dBm  IP3=inf dBm  P1dB=inf dBm  Psat=inf dBm  Gcomp=inf dBm  InternalGrounding=on  SourceFreq=Extracted from data source  PlotFreq=[1e9:1e6:3e9] Hz  PlotType=X-Y plane  YParam1=S(1,1)  YFormat1=Magnitude (dB)  YParam2=None  YFormat2=Magnitude (dB)  YOption=Linear  XOption=Linear  SparamRepresentation=Time domain (rationalfit)  FitTol=-40  FitOpt=Fit individually  MaxPoles=48  AutoImpulseLength=on  ImpulseLength=1e-10 s  MagModeling=off  AddNoise=on  NoiseType=Noise figure  NoiseDist=White  NF=0.2  MinNF=0  Gopt=0  RN=0  CarrierFreq=0 Hz  NoiseAutoImpulseLength=on  NoiseImpulseLength=1e-10 s  ConstS21NL=on  OpFreq=0 Hz  SetOpFreqAsMaxS21=on
  IQ Modulator : simrfV2systems/IQ Modulator  classname=iqmod  Source_linear_gain=Available power gain  linear_gain=10*log10(2) dB  Poly_Coeffs=[0 1]  LOFreq=RF Hz  Zin=50  Zout=50  AddIRFilters=off  AddCSFilter=on  InternalGrounding=on  ForceNextInit=off  NFloor=-inf  GainMismatch=0 dB  PhaseMismatch=0 deg  Isolation=inf dB  AddPhaseNoise=off  PhaseNoiseOffset=1e6  PhaseNoiseLevel=-140  AutoImpulseLengthPN=on  ImpulseLengthPN=1e-10  ImpulseLength_unitPN=s  Source_Poly=Even and odd order  IPType=Input  IP2=inf dBm  IP3=inf dBm  P1dB=inf dBm  Psat=inf dBm  Gcomp=inf dBm  DesignMethodIR=Ideal  ResponseTypeIR=Lowpass  ImplementationIR=LC Tee  ImplementationIdealIR=Constant per carrier  ImplementationRationalIR=Transfer function  UseFilterOrderIR=on  FilterOrderIR=3  PassFreq_lpIR=1  PassFreq_lp_unitIR=GHz  PassFreq_hpIR=2  PassFreq_hp_unitIR=GHz  PassFreq_bpIR=[2 3]  PassFreq_bp_unitIR=GHz  PassFreq_bsIR=[1 4]  PassFreq_bs_unitIR=GHz  PassAttenIR=10*log10(2)  StopFreq_lpIR=2  StopFreq_lp_unitIR=GHz  StopFreq_hpIR=1  StopFreq_hp_unitIR=GHz  StopFreq_bpIR=[1.5 3.5]  StopFreq_bp_unitIR=GHz  StopFreq_bsIR=[2.1 2.9]  StopFreq_bs_unitIR=GHz  StopAttenIR=40  RsrcIR=50  RloadIR=50  AutoImpulseLengthIR=on  ImpulseLengthIR=1e-10  ImpulseLength_unitIR=s  DesignMethodCS=Ideal  ResponseTypeCS=Highpass  ImplementationCS=LC Tee  ImplementationIdealCS=Constant per carrier  ImplementationRationalCS=Transfer function  UseFilterOrderCS=on  FilterOrderCS=3  PassFreq_lpCS=1  PassFreq_lp_unitCS=GHz  PassFreq_hpCS=HPF_cutoff  PassFreq_hp_unitCS=Hz  PassFreq_bpCS=[2 3]  PassFreq_bp_unitCS=GHz  PassFreq_bsCS=[1 4]  PassFreq_bs_unitCS=GHz  PassAttenCS=10*log10(2)  StopFreq_lpCS=2  StopFreq_lp_unitCS=GHz  StopFreq_hpCS=1  StopFreq_hp_unitCS=GHz  StopFreq_bpCS=[1.5 3.5]  StopFreq_bp_unitCS=GHz  StopFreq_bsCS=[2.1 2.9]  StopFreq_bs_unitCS=GHz  StopAttenCS=40  RsrcCS=50  RloadCS=50  AutoImpulseLengthCS=on  ImpulseLengthCS=1e-10  ImpulseLength_unitCS=s
  R2 : simrfV2elements/R  classname=resistor  Resistance=50 Ohm  AddNoise=on
  R3 : simrfV2elements/R  classname=resistor  Resistance=50 Ohm  AddNoise=on
  1+ : PMIOPort  Side=Left
  Out+ : PMIOPort  Port=2  Side=Right
  1+1 : PMIOPort  Port=3  Side=Left
  connections:
  Out+/RConn1 -- IQ Modulator/RConn1
  IQ Modulator/LConn2 -- AmplifierQ/RConn1
  AmplifierI/LConn1 -- R3/RConn1
  AmplifierI/RConn1 -- IQ Modulator/LConn1
  R3/LConn1 -- 1+/RConn1
  AmplifierQ/LConn1 -- R2/RConn1
  R2/LConn1 -- 1+1/RConn1

== matlab function singleDPD/Calculate TX EVM/MATLAB Function ==
  data: rxSig input; scaledSig output; ref input; gain output
function [scaledSig, gain] = scaleRotate(rxSig,ref)
persistent c
persistent invCov
if isempty(c)
    c = complex(ones(size(rxSig)));
end
if isempty(invCov)
    invCov = complex(ones(size(rxSig)));
end

scaledSig = c.*rxSig;
errsig = ref - scaledSig;

% RLS algorithm
lambda = 0.99;
XP = conj(rxSig).*invCov;
invDen = 1./(lambda + XP.*rxSig);
K = invDen.*(invCov.*rxSig);
invCov = (1/lambda)*(invCov - K.*XP);
c = c + errsig .* conj(K);

gain = c;
